simulink library "dsplinalg"  (Simulink 3.00)
libraries: dsplinalg x10, dspmtrx2 x4
settings Model: RequirementInfo=9  Creator=tbryan  LastModifiedBy=jeff

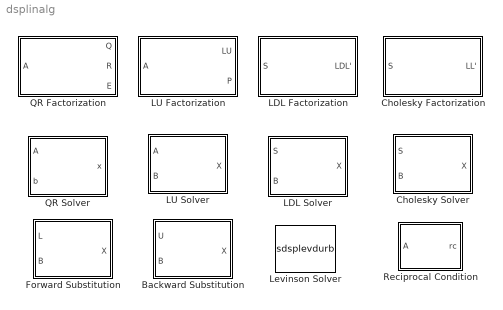
== system dsplinalg ==
  Backward Substitution : Subsystem  mask(Backward Substitution){unit=off}
      mask prompts: unit "Force input to be unit-upper triangular"
      mask help: Solve UX=B where U is an upper (or unit-upper) triangular matrix. U must be square. B must have the same number of rows as U.
      mask init:
      | x=[ 0.45 0.45 0.18 0.45 NaN 0.495 0.585 0.585 0.495 0.495 NaN 0.63 0.675 NaN 0.63 0.675 NaN 0.72 0.81 0.81 0.72 0.72 ];
      | y=[ 0.1 0.7 0.7 0.1 NaN 0.1 0.1 0.7 0.7 0.1 NaN 0.35 0.35 NaN 0.45 0.45 NaN 0.1 0.1 0.7 0.7 0.1 ];
      mask Help: web(dspbhelp);
      mask Display: plot(x,y); text(.4,0.9,'U X = B')
  Cholesky Factorization : Subsystem  mask(Cholesky Factorization){errmode=Warning}
      mask prompts: errmode "Invalid input matrix:"
      mask help: Uses only the diagonal and the upper triangle of S. The lower triangle is assumed to be the (complex conjugate) transpose of the upper. Only for use with a symmetric (Hermitian) positive definite input matrix S. Input must be square.
      mask init:
      | x=[0.5336 0.782 0.5336 0.5336 NaN 0.8234 0.575 0.8234 0.8234 NaN 0.1104 0.414 0.414 0.1104 0.1104 NaN 0.1104 0.414 NaN 0.483 0.483 0.437 0.437 0.483 0.483 0.5198 0.483];
      | y=[0.142 0.142 0.694 0.142 NaN 0.142 0.694 0.694 0.142 NaN 0.142 0.142 0.694 0.694 0.142 NaN 0.694 0.142 NaN 0.3582 0.395 0.395 0.441 0.441 0.4778 0.418 0.3582];
      mask Help: web(dspbhelp);
      mask StyleString: popup(Ignore|Warning|Error)
      mask Display:
      | plot(x,y);
      | text(.3,0.9,'S = LL''')
  Cholesky Solver : Subsystem  mask(Cholesky Solver){errmode=Warning}
      mask prompts: errmode "Invalid input matrix:"
      mask help: Solve SX=B using Cholesky factorization. S must be a square, symmetric (Hermitian) positive definite matrix. B must have the same number of rows as S.
      mask init:
      | x=[ 0.135 0.475 .475 0.135 0.135 NaN .135 .475 NaN 0.55 0.64 0.64 0.55 0.55 NaN 0.685 0.73 NaN 0.685 0.73 NaN 0.775 0.865 0.865 0.775 0.775 ];
      | y=[ 0.1 0.1 0.7 0.7 .1 NaN .7 .1 NaN 0.1 0.1 0.7 0.7 0.1 NaN 0.35 0.35 NaN 0.45 0.45 NaN 0.1 0.1 0.7 0.7 0.1 ];
      | set_param([gcb '/Cholesky'],'errmode',errmode);
      mask Help: web(dspbhelp);
      mask StyleString: popup(Ignore|Warning|Error)
      mask Display:
      | plot(x,y);
      | text(.17,0.9,'SX=B (Chol)')
  Forward Substitution : Subsystem  mask(Forward Substitution){unit=off}
      mask prompts: unit "Force input to be unit-lower triangular"
      mask help: Solve LX=B where L is a lower (or unit-lower) triangular matrix. L must be square. B must have the same number of rows as L.
      mask init:
      | x=[ 0.18 0.45 0.18 0.18 NaN 0.495 0.585 0.585 0.495 0.495 NaN 0.63 0.675 NaN 0.63 0.675 NaN 0.72 0.81 0.81 0.72 0.72 ];
      | y=[ 0.1 0.1 0.7 0.1 NaN 0.1 0.1 0.7 0.7 0.1 NaN 0.35 0.35 NaN 0.45 0.45 NaN 0.1 0.1 0.7 0.7 0.1 ];
      mask Help: web(dspbhelp);
      mask Display: plot(x,y); text(.4,0.9,'L X = B')
  LDL Factorization : Subsystem  mask(LDL Factorization){}
      mask help: Uses only the diagonal and the upper triangle of S. Only for use with a symmetric (Hermitian) positive definite input matrix S. Input must be square. Stores L (a unit-lower triangle), U (a unit-upper triangle) and D (a diagonal matrix) in the output matrix.
      mask init:
      | x=[0.47991 0.64515 0.47991 0.47991 NaN 0.74919 0.58395 0.74919 0.74919 NaN 0.694875 0.52275 NaN 0.1173 0.36975 0.36975 0.1173 0.1173 NaN 0.1173 0.36975 NaN 0.427125 0.427125 0.388875 0.388875 0.427125 0.427125 0.457725 0.427125];
      | y=[0.185 0.185 0.695 0.185 NaN 0.185 0.695 0.695 0.185 NaN 0.185 0.695 NaN 0.185 0.185 0.695 0.695 0.185 NaN 0.695 0.185 NaN 0.38475 0.41875 0.41875 0.46125 0.46125 0.49525 0.44 0.38475];
      mask Help: web(dspbhelp);
      mask Display:
      | plot(x,y);
      | text(.25,0.9,'S = L D L''')
  LDL Solver : Subsystem  mask(LDL Solver){}
      mask help: Solve Sx=b using LDL' factorization. Only for use with a symmetric (Hermitian) positive definite input matrix S. Input must be square.
      mask init:
      | Bcols=1;
      | x=[ 0.135 0.475 .475 0.135 0.135 NaN .135 .475 NaN 0.55 0.64 0.64 0.55 0.55 NaN 0.685 0.73 NaN 0.685 0.73 NaN 0.775 0.865 0.865 0.775 0.775 ];
      | y=[ 0.1 0.1 0.7 0.7 0.1 NaN .7 .1 NaN 0.1 0.1 0.7 0.7 0.1 NaN 0.35 0.35 NaN 0.45 0.45 NaN 0.1 0.1 0.7 0.7 0.1 ];
      mask Help: web(dspbhelp);
      mask Display:
      | plot(x,y);
      | text(.25,0.9,'Sx=b (LDL'')')
  LU Factorization : Subsystem  mask(LU Factorization){}
      mask help: LU factorization with row pivoting. Stores L (a unit-lower triangular matrix) in the lower triangle and U in the upper triangle of the output matrix. Permutation vector P is output separately. Input must be square.
      mask init:
      | x=[ 0.58 0.85 0.58 0.58 NaN 0.895 0.625 0.895 0.895 NaN 0.12 0.45 0.45 0.12 0.12 NaN 0.525 0.525 0.475 0.475 0.525 0.525 0.565 0.525 ];
      | y=[ 0.1 0.1 0.7 0.1 NaN 0.1 0.7 0.7 0.1 NaN 0.1 0.1 0.7 0.7 0.1 NaN 0.335 0.375 0.375 0.425 0.425 0.465 0.4 0.335 ];
      mask Help: web(dspbhelp);
      mask Display: plot(x,y); text(.25,0.9,'P A = L U')
  LU Solver : Subsystem  mask(LU Solver){}
      mask help: Solve Ax=b using LU decomposition. Input must be square.
      mask init:
      | Bcols=1;
      | x=[ 0.135 .475 0.475 0.135 .135 NaN 0.55 0.64 0.64 0.55 0.55 NaN 0.685 0.73 NaN 0.685 0.73 NaN 0.775 0.865 0.865 0.775 0.775 ];
      | y=[ 0.1 0.1 0.7 0.7 0.1 NaN 0.1 0.1 0.7 0.7 0.1 NaN 0.35 0.35 NaN 0.45 0.45 NaN 0.1 0.1 0.7 0.7 0.1 ];
      mask Help: web(dspbhelp);
      mask Display:
      | plot(x,y);
      | text(.3,0.9,'Ax=b (LU)')
  Levinson Solver : S-Function  FunctionName=sdsplevdurb  Parameters=fcn,otype  PortCounts=[]  mask(Levinson Solver){fcn=A and K, otype=on}
      mask prompts: fcn "Output(s):"; otype "Special-case handling of zero input"
      mask help: Solve Hermitian Toeplitz system of equations using the Levinson-Durbin recursion. Input is typically a vector of autocorrelation coefficients with lag 0 as the first element. Outputs polynomial coefficients A and/or reflection coefficients K.
      mask init:
      | s = dspblklevdurb(fcn);
      mask Help: web(dspbhelp);
      mask StyleString: popup(A and K|A|K),checkbox
      mask Display:
      | disp('L-D');
      | port_label('input',s.i1,s.i1s);
      | port_label('input',s.i2,s.i2s);
      | port_label('output',s.o1,s.o1s);
      | port_label('output',s.o2,s.o2s);
  QR Factorization : Subsystem  mask(QR Factorization){Acols=5}
      mask prompts: Acols "Columns in A:"
      mask help: QR factorization with column pivoting. Q is a unitary matrix, R is an upper triangular matrix (U), and E is a permutation vector such that A(:,E) = Q*R.
      mask init:
      | x=[ 0.4785 0.6699 0.6699 0.4785 0.4785 NaN 0.875568 0.70644 0.875568 0.875568 NaN 0.12006 0.348 0.348 0.12006 0.12006 NaN 0.424125 0.424125 0.384975 0.384975 0.424125 0.424125 0.455445 0.424125 ];
      | y=[ 0.1 0.1 .7 0.7 0.1 NaN 0.1 0.7 0.7 0.1 NaN 0.1 0.1 0.7 0.7 0.1 NaN 0.335 0.375 0.375 0.425 0.425 0.465 0.4 0.335 ];
      mask Help: web(dspbhelp);
      mask Display:
      | plot(x,y);
      | text(.2,0.9,'A(:,E) = Q R')
  QR Solver : Subsystem  mask(QR Solver){}
      mask help: Solve Ax=b using QR factorization.
      mask init:
      | x=[ 0.135 0.475 .475 0.135 0.135 NaN 0.55 0.64 0.64 0.55 0.55 NaN 0.685 0.73 NaN 0.685 0.73 NaN 0.775 0.865 0.865 0.775 0.775 ];
      | y=[ 0.1 0.1 0.7 0.7 0.1 NaN 0.1 0.1 0.7 0.7 0.1 NaN 0.35 0.35 NaN 0.45 0.45 NaN 0.1 0.1 0.7 0.7 0.1 ];
      mask Help: web(dspbhelp);
      mask Display:
      | plot(x,y);
      | text(.25,0.9,'Ax=b (QR)')
  Reciprocal Condition : Subsystem
      mask Type: Reciprocal Condition
      mask Description: Estimates the reciprocal of the condition of a square input matrix in the 1-norm.  If input is well conditioned, the output is near 1.0.  If input is badly conditioned, output is near 0.0.
      mask Help: web(dspbhelp);
      mask Display: disp('RCond')

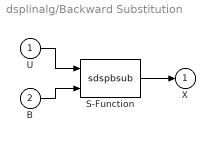
== system dsplinalg/Backward Substitution ==
  U : Inport  Port=1
  B : Inport  Port=2
  S-Function : S-Function  FunctionName=sdspbsub  Parameters=unit  PortCounts=[]
  X : Outport  Port=1  InitialOutput=0
  wires:
  S-Function/1 -> X/1
  U/1 -> S-Function/1
  B/1 -> S-Function/2

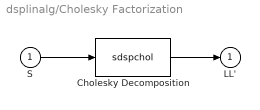
== system dsplinalg/Cholesky Factorization ==
  S : Inport  Port=1
  Cholesky Decomposition : S-Function  FunctionName=sdspchol  Parameters=errmode  PortCounts=[]
  LL' : Outport  Port=1  InitialOutput=0
  wires:
  S/1 -> Cholesky Decomposition/1
  Cholesky Decomposition/1 -> LL'/1

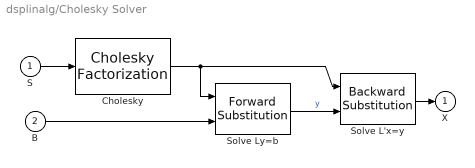
== system dsplinalg/Cholesky Solver ==
  S : Inport  Port=1
  B : Inport  Port=2
  Cholesky : dsplinalg/Cholesky Factorization  errmode=Warning
  Solve L'x=y : dsplinalg/Backward Substitution  unit=off
  Solve Ly=b : dsplinalg/Forward Substitution  unit=off
  X : Outport  Port=1  InitialOutput=0
  wires:
  S/1 -> Cholesky/1
  Solve Ly=b/1 -> Solve L'x=y/2  "y"
  Solve L'x=y/1 -> X/1
  B/1 -> Solve Ly=b/2
  Cholesky/1 -> Solve Ly=b/1, Solve L'x=y/1

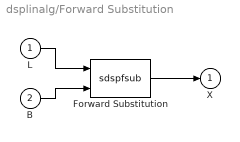
== system dsplinalg/Forward Substitution ==
  L : Inport  Port=1
  B : Inport  Port=2
  Forward Substitution : S-Function  FunctionName=sdspfsub  Parameters=unit  PortCounts=[]
  X : Outport  Port=1  InitialOutput=0
  wires:
  B/1 -> Forward Substitution/2
  L/1 -> Forward Substitution/1
  Forward Substitution/1 -> X/1

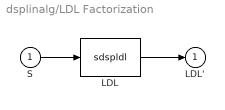
== system dsplinalg/LDL Factorization ==
  S : Inport  Port=1
  LDL : S-Function  FunctionName=sdspldl  PortCounts=[]
  LDL' : Outport  Port=1  InitialOutput=0
  wires:
  S/1 -> LDL/1
  LDL/1 -> LDL'/1

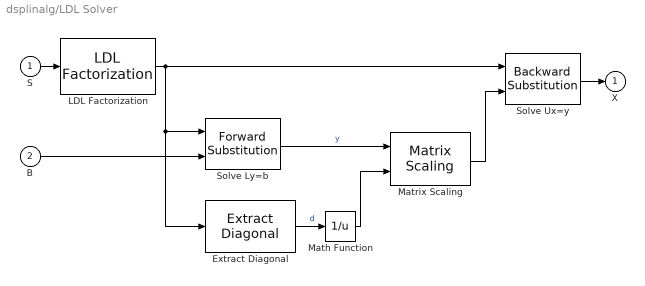
== system dsplinalg/LDL Solver ==
  S : Inport  Port=1
  B : Inport  Port=2
  Extract Diagonal : dspmtrx2/Extract Diagonal  ncols=-1
  LDL Factorization : dsplinalg/LDL Factorization
  Math Function : Math  Operator=reciprocal  OutputSignalType=auto
  Matrix Scaling : dspmtrx2/Matrix Scaling  mode=Scale Rows (D*A)  cols=Bcols
  Solve Ly=b : dsplinalg/Forward Substitution  unit=on
  Solve Ux=y : dsplinalg/Backward Substitution  unit=on
  X : Outport  Port=1  InitialOutput=0
  wires:
  Solve Ux=y/1 -> X/1
  LDL Factorization/1 -> Solve Ux=y/1, Solve Ly=b/1, Extract Diagonal/1
  B/1 -> Solve Ly=b/2
  S/1 -> LDL Factorization/1
  Solve Ly=b/1 -> Matrix Scaling/1  "y"
  Matrix Scaling/1 -> Solve Ux=y/2
  Extract Diagonal/1 -> Math Function/1  "d"
  Math Function/1 -> Matrix Scaling/2

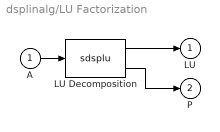
== system dsplinalg/LU Factorization ==
  A : Inport  Port=1
  LU Decomposition : S-Function  FunctionName=sdsplu  PortCounts=[]
  LU : Outport  Port=1  InitialOutput=0
  P : Outport  Port=2  InitialOutput=0
  wires:
  LU Decomposition/2 -> P/1
  A/1 -> LU Decomposition/1
  LU Decomposition/1 -> LU/1

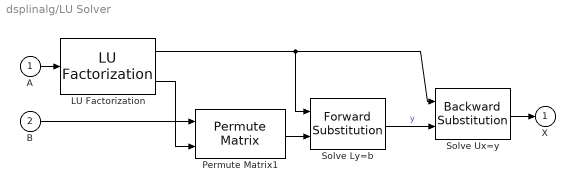
== system dsplinalg/LU Solver ==
  A : Inport  Port=1
  B : Inport  Port=2
  LU Factorization : dsplinalg/LU Factorization
  Permute Matrix1 : dspmtrx2/Permute Matrix  mode=Rows  errmode=Clip Index  cols=Bcols
  Solve Ly=b : dsplinalg/Forward Substitution  unit=on
  Solve Ux=y : dsplinalg/Backward Substitution  unit=off
  X : Outport  Port=1  InitialOutput=0
  wires:
  A/1 -> LU Factorization/1
  Permute Matrix1/1 -> Solve Ly=b/2
  Solve Ux=y/1 -> X/1
  Solve Ly=b/1 -> Solve Ux=y/2  "y"
  B/1 -> Permute Matrix1/1
  LU Factorization/2 -> Permute Matrix1/2
  LU Factorization/1 -> Solve Ly=b/1, Solve Ux=y/1

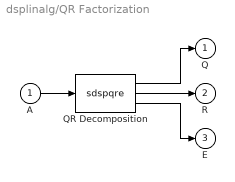
== system dsplinalg/QR Factorization ==
  A : Inport  Port=1
  QR Decomposition : S-Function  FunctionName=sdspqre  Parameters=Acols  PortCounts=[]
  Q : Outport  Port=1  InitialOutput=0
  R : Outport  Port=2  InitialOutput=0
  E : Outport  Port=3  InitialOutput=0
  wires:
  A/1 -> QR Decomposition/1
  QR Decomposition/1 -> Q/1
  QR Decomposition/2 -> R/1
  QR Decomposition/3 -> E/1

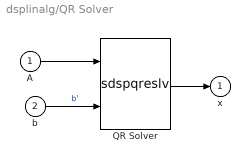
== system dsplinalg/QR Solver ==
  A : Inport  Port=1
  b : Inport  Port=2
  QR Solver : S-Function  FunctionName=sdspqreslv  PortCounts=[]
  x : Outport  Port=1  InitialOutput=0
  wires:
  QR Solver/1 -> x/1
  A/1 -> QR Solver/1
  b/1 -> QR Solver/2  "b'"

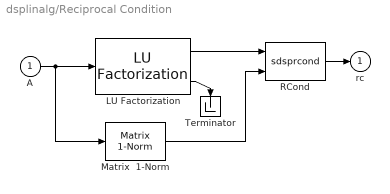
== system dsplinalg/Reciprocal Condition ==
  A : Inport  Port=1
  LU Factorization : dsplinalg/LU Factorization
  Matrix  1-Norm : dspmtrx2/Matrix  1-Norm  Cols=-1
  RCond : S-Function  FunctionName=sdsprcond  PortCounts=[]
  Terminator : Terminator
      settings: Orientation=down
  " rc" : Outport  Port=1  InitialOutput=0
  wires:
  A/1 -> Matrix  1-Norm/1, LU Factorization/1
  Matrix  1-Norm/1 -> RCond/2
  RCond/1 -> " rc"/1
  LU Factorization/1 -> RCond/1
  LU Factorization/2 -> Terminator/1
